simulink model "calc"  (R2018b)
settings: Solver=FixedStepDiscrete  StartTime=0.0  StopTime=10.0  RelTol=1e-3
settings Model: Creator=lenovo2  LastModifiedBy=lenovo2
settings OptimizationCC: DefaultParameterBehavior=Inlined  EnhancedBackFolding=on  PassReuseOutputArgsAs=Individual arguments  OptimizeBlockOrder=speed  DifferentSizesBufferReuse=on  OptimizationCustomize=off
settings DebuggingCC: UnderspecifiedInitializationDetection=Classic  MergeDetectMultiDrivingBlocksExec=none  ParameterTunabilityLossMsg=error
settings ModelReferenceCC: PropagateSignalLabelsOutOfModel=off
settings SFSimCC: MATLABDynamicMemAlloc=off
settings RTWCC: SystemTargetFile=ert.tlc  GenCodeOnly=on  TemplateMakefile=ert_default_tmf  GenerateReport=on  IncludeHyperlinkInReport=on  LaunchReport=on  GenerateTraceInfo=on  GenerateTraceReport=on  GenerateTraceReportSl=on  GenerateTraceReportSf=on  GenerateTraceReportEml=on
settings CodeAppCC: ForceParamTrailComments=on  IgnoreCustomStorageClasses=off  OperatorAnnotations=on  SimulinkDataObjDesc=on  SFDataObjDesc=on  InsertBlockDesc=on
settings ERTTargetCC: TargetLangStandard=C99 (ISO)  GenerateSampleERTMain=on  InlinedParameterPlacement=NonHierarchical  ERTCustomFileTemplate=example_file_process.tlc

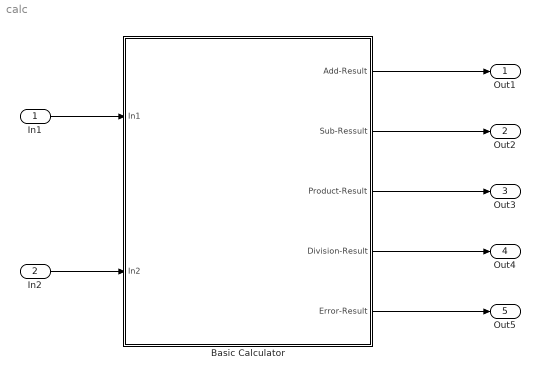
== system calc ==
  In1 : Inport
  In2 : Inport  Port=2
  Basic Calculator : Subsystem  TreatAsAtomicUnit=on
      settings: MinAlgLoopOccurrences=on  RTWFcnNameOpts=Use subsystem name
  Out1 : Outport
  Out2 : Outport  Port=2
  Out3 : Outport  Port=3
  Out4 : Outport  Port=4
  Out5 : Outport  Port=5
  wires:
  In1/1 -> Basic Calculator/1(In1)
  Basic Calculator/4(Division-Result) -> Out4/1
  Basic Calculator/3(Product-Result) -> Out3/1
  Basic Calculator/1(Add-Result) -> Out1/1
  Basic Calculator/2(Sub-Ressult) -> Out2/1
  Basic Calculator/5("Error-Result ") -> Out5/1
  In2/1 -> Basic Calculator/2(In2)

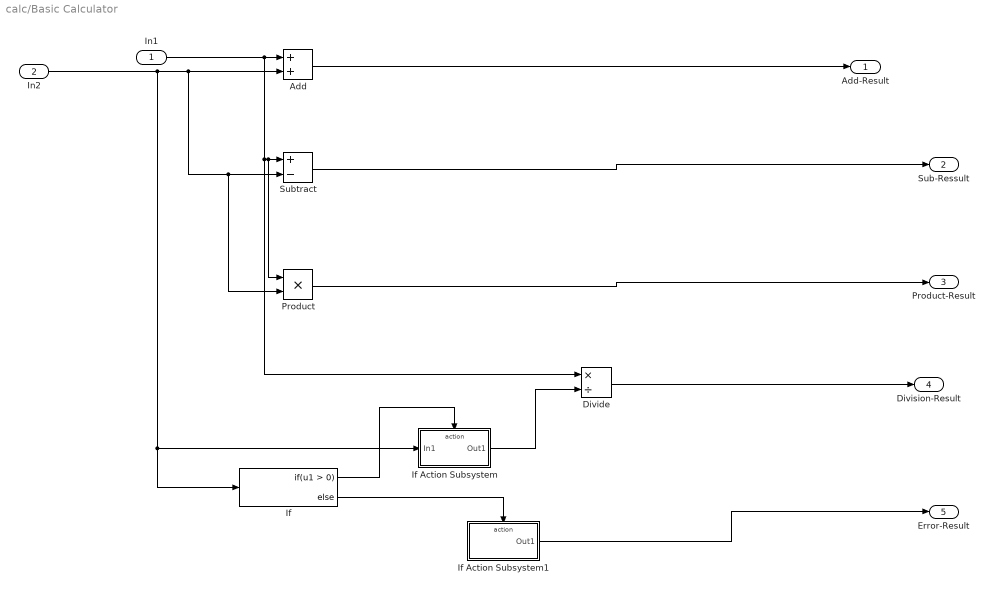
== system calc/Basic Calculator ==
  In1 : Inport
  In2 : Inport  Port=2
  Add : Sum
  Divide : Product  Inputs=*/
  If : If
  If Action Subsystem : Subsystem  TreatAsAtomicUnit=on
  If Action Subsystem1 : Subsystem  TreatAsAtomicUnit=on
  Product : Product
  Subtract : Sum  Inputs=+-
  Add-Result : Outport
  Sub-Ressult : Outport  Port=2
  Product-Result : Outport  Port=3
  Division-Result : Outport  Port=4
  "Error-Result " : Outport  Port=5
  wires:
  If Action Subsystem/1(Out1) -> Divide/2
  In1/1 -> Product/1, Subtract/1, Divide/1, Add/1
  In2/1 -> If Action Subsystem/1(In1), If/1, Product/2, Subtract/2, Add/2
  Add/1 -> Add-Result/1
  If/2 -> If Action Subsystem1/Action
  If/1 -> If Action Subsystem/Action
  Subtract/1 -> Sub-Ressult/1
  Product/1 -> Product-Result/1
  Divide/1 -> Division-Result/1
  If Action Subsystem1/1(Out1) -> "Error-Result "/1

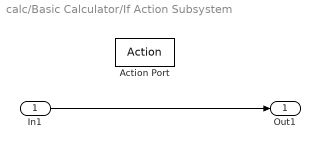
== system calc/Basic Calculator/If Action Subsystem ==
  In1 : Inport
  Action Port : ActionPort  ActionType=then
  Out1 : Outport
  wires:
  In1/1 -> Out1/1

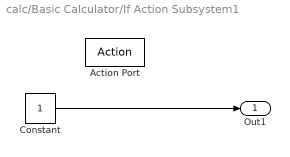
== system calc/Basic Calculator/If Action Subsystem1 ==
  Action Port : ActionPort  ActionType=else
  Constant : Constant  OutDataTypeStr=uint8
  Out1 : Outport
  wires:
  Constant/1 -> Out1/1
